simulink model "BESS_F_V_Controle"  (R2017b)
settings: Solver=ode45  StartTime=0.0  StopTime=10  RelTol=1e-3  EnableMultiTasking=on
values from neighbouring files (symbols this model uses):
  beta = beta (k)    [Parameter_2M_DFIG_BESS.m]
  Cbus = 80e-3    (= 0.08)    [Parameter_2M_DFIG_BESS.m]
  Cbus_bess = 15e-3    (= 0.015)    [Parameter_2M_DFIG_BESS.m]
  Cfilter = 80e-3    (= 0.08)    [Parameter_2M_DFIG_BESS.m]
  cp_opt_abs = abs(max(Cp))    [Parameter_2M_DFIG_BESS.m]
  D = 0.1    [Parameter_2M_DFIG_BESS.m]
  f = 60    [Parameter_2M_DFIG_BESS.m]
  Fs = 1.8    [Parameter_2M_DFIG_BESS.m]
  fsw = 4e3    (= 4000)    [Parameter_2M_DFIG_BESS.m]
  J = 90    [Parameter_2M_DFIG_BESS.m]
  ki_id = (wni^2)*Lr*sigma    (= 491.599501999)    [Parameter_2M_DFIG_BESS.m]
  ki_idg = (wnig^2)*Lg    (= 68.6450725305)    [Parameter_2M_DFIG_BESS.m]
  ki_iq = ki_id    (= 491.599501999)    [Parameter_2M_DFIG_BESS.m]
  ki_iqg = ki_idg    (= 68.6450725305)    [Parameter_2M_DFIG_BESS.m]
  ki_v = -300000    [Parameter_2M_DFIG_BESS.m]
  kp_id = (2*wni*sigma*Lr)-Rr    (= 0.5771)    [Parameter_2M_DFIG_BESS.m]
  kp_idg = (2*wnig*Lg)-Rg    (= 0.364153420404)    [Parameter_2M_DFIG_BESS.m]
  kp_iq = kp_id    (= 0.5771)    [Parameter_2M_DFIG_BESS.m]
  kp_iqg = kp_idg    (= 0.364153420404)    [Parameter_2M_DFIG_BESS.m]
  kp_v = -1000    [Parameter_2M_DFIG_BESS.m]
  Kpg = 1/(1.5*Vs*sqrt(2/3))    [Parameter_2M_DFIG_BESS.m]
  Kqg = -Kpg    [Parameter_2M_DFIG_BESS.m]
  lambda_opt = abs(lambda(posicion))    [Parameter_2M_DFIG_BESS.m]
  Lfilter = 483e-6    (= 0.000483)    [Parameter_2M_DFIG_BESS.m]
  Lg = 483e-6    (= 0.000483)    [Parameter_2M_DFIG_BESS.m]
  Lm = 2.5e-3    (= 0.0025)    [Parameter_2M_DFIG_BESS.m]
  Lr = Lm + Lsr    (= 0.002587)    [Parameter_2M_DFIG_BESS.m]
  Ls = Lm + Lsi    (= 0.002587)    [Parameter_2M_DFIG_BESS.m]
  Lsi = 87e-6    (= 8.7e-05)    [Parameter_2M_DFIG_BESS.m]
  N = 100    [Parameter_2M_DFIG_BESS.m]
  p = 2    [Parameter_2M_DFIG_BESS.m]
  Ps = 2e6    (= 2000000)    [Parameter_2M_DFIG_BESS.m]
  Radio = 44    [Parameter_2M_DFIG_BESS.m]
  Rfilter = 20e-3    (= 0.02)    [Parameter_2M_DFIG_BESS.m]
  Rg = 20e-6    (= 2e-05)    [Parameter_2M_DFIG_BESS.m]
  ro = 1.225    [Parameter_2M_DFIG_BESS.m]
  Rr = 2.9e-3    (= 0.0029)    [Parameter_2M_DFIG_BESS.m]
  Rs = 2.6e-3    (= 0.0026)    [Parameter_2M_DFIG_BESS.m]
  sigma = 1- Lm^2/(Ls*Lr)    (= 0.0661284179513)    [Parameter_2M_DFIG_BESS.m]
  Ts = 1/fsw/f    (= 4.16666666667e-06)    [Parameter_2M_DFIG_BESS.m]
  Vbus_ref = 1200    [Parameter_2M_DFIG_BESS.m]
  Vs = 690    [Parameter_2M_DFIG_BESS.m]
undefined symbols (not defined in the file or in its folder): D1, D11, Delta, DiscIntNeverNeededParam, Ion, Lithium, sigbuilder_block
libraries: powerlib x72, powerlib_meascontrol x37, electricdrivelib x1, simulink x1, sps_avr x1
(part 2 of 3)

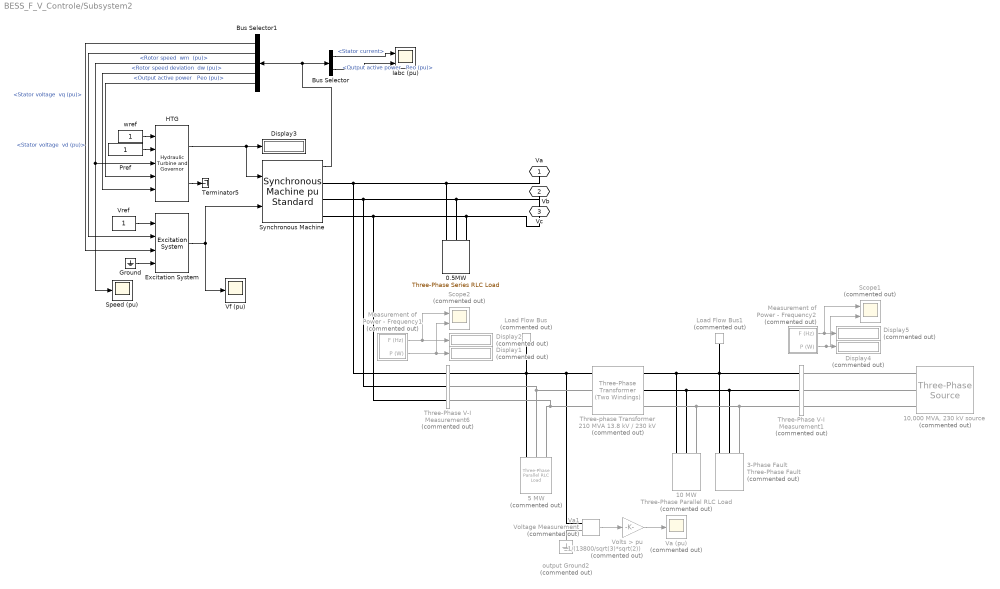
== system BESS_F_V_Controle/Subsystem2 ==
  " Iabc (pu)" : Scope  NumInputPorts=2
  " Speed (pu)" : Scope
  0.5MW : powerlib/Elements/Three-Phase Series RLC Load  LConnTagsString=A|B|C  Configuration=Y (grounded)  NominalVoltage=13800  Vabc=[1e3 1e3 1e3]  Vabcp=[1e3 1e3 1e3]  NominalFrequency=f  UnbalancedPower=off  ActivePower=0.5e6  InductivePower=0  CapacitivePower=0  Pabc=[10e3 9e3 11e3]  QLabc=[100 90 110]  QCabc=[100 90 110]  Pabcp=[10e3 9e3 11e3]  QLabcp=[100 90 110]  QCabcp=[100 90 110]  Measurements=None  LoadType=constant Z
  10 MW : powerlib/Elements/Three-Phase Parallel RLC Load  Commented=on  LConnTagsString=A|B|C  Configuration=Y (grounded)  NominalVoltage=230e3  Vabc=[1e3 1e3 1e3]  Vabcp=[1e3 1e3 1e3]  NominalFrequency=f  UnbalancedPower=off  ActivePower=10000000  InductivePower=0  CapacitivePower=0  Pabc=[10e3 9e3 11e3]  QLabc=[100 90 110]  QCabc=[100 90 110]  Pabcp=[10e3 9e3 11e3]  QLabcp=[100 90 110]  QCabcp=[100 90 110]  Measurements=None  LoadType=constant Z
  "10,000 MVA, 230 kV source" : powerlib/Electrical Sources/Three-Phase Source  Commented=on  InternalConnection=Yg  VoltagePhases=off  Voltage=(230000)*1.00006  PhaseAngle=-0.77547  Voltage_phases=[25e3 25e3 25e3]/sqrt(3)  PhaseAngles_phases=[0 -120 +120]  Frequency=60  NonIdealSource=on  SpecifyImpedance=on  Resistance=0.529  Inductance=0.0140  ShortCircuitLevel=10000e6  BaseVoltage=230e3  XRratio=10  BusType=swing  Pref=0  Qref=0  Prefabc=[10e3, 10e3, 10e3]  Qrefabc=[0, 0, 0]  Qmin=-Inf  Qmax=Inf
  3-Phase Fault : powerlib/Elements/Three-Phase Fault  Commented=on  InitialStates=0  FaultA=on  FaultB=on  FaultC=on  GroundFault=on  SwitchTimes=[ 0.1 0.2]  External=off  SwitchStatus=NaN  FaultResistance=1e-3  GroundResistance=1e-3  SnubberResistance=inf  SnubberCapacitance=inf  Measurements=None
  5 MW : powerlib/Elements/Three-Phase Parallel RLC Load  Commented=on  LConnTagsString=A|B|C  Configuration=Y (grounded)  NominalVoltage=13.8e3  Vabc=[1e3 1e3 1e3]  Vabcp=[1e3 1e3 1e3]  NominalFrequency=60  UnbalancedPower=off  ActivePower=5000000  InductivePower=0  CapacitivePower=0  Pabc=[10e3 9e3 11e3]  QLabc=[100 90 110]  QCabc=[100 90 110]  Pabcp=[10e3 9e3 11e3]  QLabcp=[100 90 110]  QCabcp=[100 90 110]  Measurements=None  LoadType=constant Z
  Bus Selector : BusSelector  OutputSignals="Stator current,Output active power   Peo (pu)"
  Bus Selector1 : BusSelector  OutputSignals="dq0 components.Stator voltage  vq (pu),dq0 components.Stator voltage  vd (pu),Mechanical.Rotor speed  wm  (pu),Mechanical.Rotor speed deviation  dw (pu),Output active power   Peo (pu)"
  Display{1..2,4..5} (4 alike) : Display  Commented=on
  Display3 : Display
  Excitation System : sps_avr/Excitation System  tr=20e-3  reg=[ 300, 0.001 ]  exc=[ 1, 0 ]  tgr=[ 0, 0 ]  damp=[ 0.001, 0.1 ]  sat=[ 0, 0 ]  lim=[ -11.5, 11.5, 0 ]  v0=[1,1.29071]
      settings: SourceProductName=Simscape Power Systems  SourceProductBaseCode=PS
  Ground : Ground
  HTG : powerlib/Machines/Hydraulic Turbine and Governor  sm="[ 10/3  0.07 ]"  gate="[  0.01  0.97518  -0.1  0.1 ]"  reg="[  0.05  1.163  0.105  0  0.01  ]"  hyd="[  0  2.67  ]"  dref=0  po=1
      settings: SourceProductName=Simscape Power Systems  SourceProductBaseCode=PS
  Load Flow Bus : powerlib/Measurements/Load Flow Bus  Commented=on  LConnTagsString=a  Phases=single  Connectors=on one side  ID=B1  Vbase=13.8e3  Vref=1  Vangle=0  VLF=1  VLFb=1  VLFc=1  angleLF=-23.67  angleLFb=0  angleLFc=0
      settings: AttributesFormatString=%<ID>\n%<Vbase>V\n%<VLF>pu\n%<angleLF>deg.  SourceProductName=Simscape Power Systems
  Load Flow Bus1 : powerlib/Measurements/Load Flow Bus  Commented=on  LConnTagsString=a  Phases=single  Connectors=on one side  ID=B2  Vbase=230e3  Vref=1  Vangle=0  VLF=1  VLFb=1  VLFc=1  angleLF=0  angleLFb=0  angleLFc=0
      settings: AttributesFormatString=%<ID>\n%<Vbase>V\n%<VLF>pu\n%<angleLF>deg.  SourceProductName=Simscape Power Systems
  Measurement of Power - Frequency1 : Subsystem  Commented=on
  Measurement of Power - Frequency2 : Subsystem  Commented=on
  Pref : Constant
  Scope1 : Scope  Commented=on  NumInputPorts=2
  Scope2 : Scope  Commented=on  NumInputPorts=2
  "Synchronous Machine " : powerlib/Machines/Synchronous Machine pu Standard  PresetModel=No  MechanicalLoad=Mechanical power Pm  ShowDetailedParameters=on  RotorType=Salient-pole  Units=per unit standard parameters  MeasurementBus=off  NominalParameters="[ 7.5e6  13800   f ]"  Reactances1=[ 31 32 33 34 35 36 37 ]  Reactances2=[ 1.305, 0.296, 0.252, 0.474, 0.243, 0.18 ]  dAxisTimeConstants=Short-circuit  qAxisTimeConstants=Open-circuit  TimeConstants1=[]  TimeConstants2=[]  TimeConstants3=[]  TimeConstants4=[]  TimeConstants5=[ 1.01, 0.053, 0.1 ]  TimeConstants6=[]  TimeConstants7=[]  TimeConstants8=[]  StatorResistance=2.8544e-3  Mechanical=[ 3.2 0 2]  PolePairs=2  InitialConditions=[0 -94.2826 0.750185 0.750185 0.750185 -24.943 -144.943 95.057 1.29071]  SetSaturation=off  Saturation=[0.6404,0.7127,0.8441,0.9214,0.9956,1.082,1.19,1.316,1.457;0.7,0.7698,0.8872,0.9466,0.9969,1.046,1.1,1.151,1.201]  LoadFlowParameters=[1 150000000 0 0]  TsPowergui=0  TsBlock=-1  IterativeModel=Trapezoidal non iterative  IterativeDiscreteModel=Trapezoidal non iterative  BusType=PV  Pref=150000000  Qref=0  Qmin=-Inf  Qmax=Inf  PLF=0  QLF=0
      settings: AttributesFormatString=\n\n  SourceProductName=Simscape Power Systems
  Terminator5 : Terminator
  Three-Phase V-I Measurement1 : powerlib/Measurements/Three-Phase V-I Measurement  Commented=on  VoltageMeasurement=phase-to-ground  SetLabelV=on  LabelV=V_ac_syn_low2  Vpu=off  VpuLL=off  CurrentMeasurement=yes  SetLabelI=on  LabelI=I_ac_syn_low2  Ipu=off  Pbase=100e6  Vbase=500e3  OutputType=Complex  PhasorSimulation=off  PSBequivalent=0
  Three-Phase V-I Measurement6 : powerlib/Measurements/Three-Phase V-I Measurement  Commented=on  VoltageMeasurement=phase-to-ground  SetLabelV=on  LabelV=V_ac_syn_low1  Vpu=off  VpuLL=off  CurrentMeasurement=yes  SetLabelI=on  LabelI=I_ac_syn_low1  Ipu=off  Pbase=100e6  Vbase=500e3  OutputType=Complex  PhasorSimulation=off  PSBequivalent=0
  Three-phase Transformer 210 MVA 13.8 kV / 230 kV : powerlib/Elements/Three-Phase Transformer (Two Windings)  Commented=on  Winding1Connection=Delta (D1)  Winding2Connection=Yg  CoreType=Three single-phase transformers  SetSaturation=off  Hysteresis=off  DataFile='hysteresis'  SetInitialFlux=off  Measurements=None  UNITS=pu  NominalPower=[ 210e6 60 ]  Winding1="[ 13.8e3 0.0027  0.08]"  Winding2=[ 230e3 0.0027 0.08]  Rm=500  Lm=500  L0=0.5  Saturation="[ 0,0  ;  0.005,1.2  ;  1.0,1.4 ]"  InitialFluxes=[ 0.8 , -0.8 , 0.7 ]  MoreParameters=off  BreakLoop=off  DataType=off  TransfoNumber=0
  Va (pu) : Scope  Commented=on
  Va1 : powerlib/Measurements/Voltage Measurement  Tag=PoWeRsYsTeMmEaSuReMeNt  Commented=on  PhasorSimulation=off  OutputType=Magnitude  PSBequivalent=0
  Vf (pu) : Scope
  Volts > pu : Gain  Commented=on  Gain=1/(13800/sqrt(3)*sqrt(2))  SaturateOnIntegerOverflow=on  OutDataTypeStr=Inherit: Same as input  ParamDataTypeStr=Inherit: Same as input
  Vref : Constant
  output Ground2 : powerlib/Elements/Ground  Commented=on  LConnTagsString=a
  wref : Constant
  Va : PMIOPort  Port=1  Side=Left
  Vb : PMIOPort  Port=2  Side=Left
  Vc : PMIOPort  Port=3  Side=Left
  wires:
  Bus Selector1/5 -> HTG/4  "<Output active power   Peo (pu)>"
  HTG/2 -> Terminator5/1
  Bus Selector1/3 -> HTG/3, " Speed (pu)"/1  "<Rotor speed  wm  (pu)>"
  Bus Selector/1 -> " Iabc (pu)"/1  "<Stator current>"
  Bus Selector1/2 -> Excitation System/2  "<Stator voltage  vd (pu)>"
  Ground/1 -> Excitation System/4
  Bus Selector1/1 -> Excitation System/3  "<Stator voltage  vq (pu)>"
  Va1/1 -> Volts > pu/1
  Excitation System/1 -> Vf (pu)/1, "Synchronous Machine "/2
  Bus Selector1/4 -> HTG/5  "<Rotor speed deviation  dw (pu)>"
  Volts > pu/1 -> Va (pu)/1
  Pref/1 -> HTG/2
  wref/1 -> HTG/1
  Vref/1 -> Excitation System/1
  "Synchronous Machine "/1 -> Bus Selector/1, Bus Selector1/1
  Measurement of Power - Frequency1/1(F (Hz)) -> Scope2/1, Display2/1
  Measurement of Power - Frequency1/2(P (W)) -> Scope2/2, Display1/1
  Bus Selector/2 -> " Iabc (pu)"/2  "<Output active power   Peo (pu)>"
  HTG/1 -> "Synchronous Machine "/1, Display3/1
  Measurement of Power - Frequency2/1(F (Hz)) -> Scope1/1, Display5/1
  Measurement of Power - Frequency2/2(P (W)) -> Scope1/2, Display4/1
  connections:
  Va1/LConn1 -- Three-Phase V-I Measurement6/RConn1 -- 5 MW/LConn1 -- Load Flow Bus/LConn1 -- Three-phase Transformer 210 MVA 13.8 kV / 230 kV/LConn1
  5 MW/LConn3 -- Three-Phase V-I Measurement6/RConn3 -- Three-phase Transformer 210 MVA 13.8 kV / 230 kV/LConn3
  10 MW/LConn2 -- Three-phase Transformer 210 MVA 13.8 kV / 230 kV/RConn2 -- Three-Phase V-I Measurement1/LConn2 -- 3-Phase Fault/LConn2
  Load Flow Bus1/LConn1 -- Three-phase Transformer 210 MVA 13.8 kV / 230 kV/RConn1 -- 10 MW/LConn1 -- Three-Phase V-I Measurement1/LConn1 -- 3-Phase Fault/LConn1
  3-Phase Fault/LConn3 -- Three-Phase V-I Measurement1/LConn3 -- Three-phase Transformer 210 MVA 13.8 kV / 230 kV/RConn3 -- 10 MW/LConn3
  5 MW/LConn2 -- Three-Phase V-I Measurement6/RConn2 -- Three-phase Transformer 210 MVA 13.8 kV / 230 kV/LConn2
  output Ground2/LConn1 -- Va1/LConn2
  0.5MW/LConn1 -- Three-Phase V-I Measurement6/LConn1 -- "Synchronous Machine "/RConn1 -- Va/RConn1
  Vb/RConn1 -- "Synchronous Machine "/RConn2 -- Three-Phase V-I Measurement6/LConn2 -- 0.5MW/LConn2
  0.5MW/LConn3 -- "Synchronous Machine "/RConn3 -- Three-Phase V-I Measurement6/LConn3 -- Vc/RConn1
  Three-Phase V-I Measurement1/RConn1 -- "10,000 MVA, 230 kV source"/RConn1
  Three-Phase V-I Measurement1/RConn2 -- "10,000 MVA, 230 kV source"/RConn2
  Three-Phase V-I Measurement1/RConn3 -- "10,000 MVA, 230 kV source"/RConn3

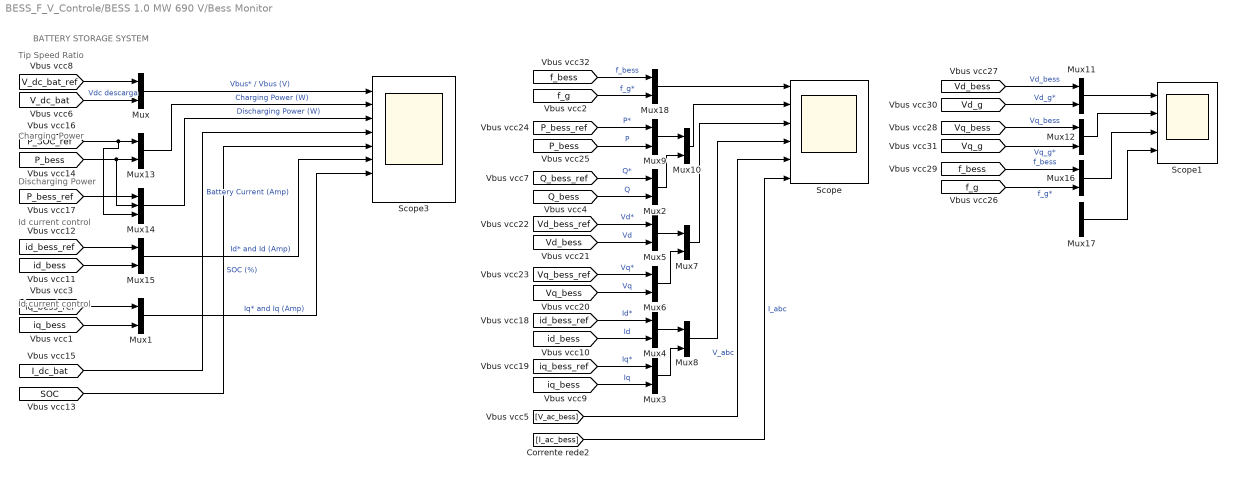
== system BESS_F_V_Controle/BESS 1.0 MW 690 V/Bess Monitor ==
  note: BATTERY STORAGE SYSTEM
  note: Tip Speed Ratio
  note: Charging Power
  note: Discharging Power
  note: Id current control
  note: Id current control
  Mux{,1..13,15..18} (18 alike) : Mux  Inputs=2
  Mux14 : Mux  Inputs=3
  Scope : Scope  NumInputPorts=6
  Scope1 : Scope  NumInputPorts=4
  Scope3 : Scope  NumInputPorts=8
  wires:
  [P_bess_ref] -> Mux14/1
  Mux13/1 -> Scope3/2  "Charging Power (W)"
  [P_SOC_ref] -> Mux14/3, Mux13/1
  [P_bess] -> Mux14/2, Mux13/2
  [id_bess_ref] -> Mux15/1
  [V_dc_bat_ref] -> Mux/1
  Mux/1 -> Scope3/1  "Vbus* / Vbus (V)"
  [id_bess] -> Mux15/2
  Mux14/1 -> Scope3/3  "Discharging Power (W)"
  [SOC] -> Scope3/5  "SOC (%)"
  [I_dc_bat] -> Scope3/4  "Battery Current (Amp)"
  Mux15/1 -> Scope3/6  "Id* and Id (Amp)"
  [V_dc_bat] -> Mux/2  "Vdc descarga"
  [iq_bess] -> Mux1/2
  [iq_bess_ref] -> Mux1/1
  Mux1/1 -> Scope3/7  "Iq* and Iq (Amp)"
  [Q_bess_ref] -> Mux2/1  "Q*"
  [Q_bess] -> Mux2/2  "Q"
  [iq_bess_ref] -> Mux3/1  "Iq*"
  [id_bess] -> Mux4/2  "Id"
  [iq_bess] -> Mux3/2  "Iq"
  [id_bess_ref] -> Mux4/1  "Id*"
  [Vq_bess_ref] -> Mux6/1  "Vq*"
  [Vq_bess] -> Mux6/2  "Vq"
  Mux4/1 -> Mux8/1
  Mux6/1 -> Mux7/2
  Mux5/1 -> Mux7/1
  Mux7/1 -> Scope/3
  Mux3/1 -> Mux8/2
  Mux8/1 -> Scope/4
  [V_ac_bess] -> Scope/5  "V_abc"
  [I_ac_bess] -> Scope/6  "I_abc"
  [P_bess_ref] -> Mux9/1  "P*"
  [P_bess] -> Mux9/2  "P"
  Mux9/1 -> Mux10/1
  Mux2/1 -> Mux10/2
  Mux10/1 -> Scope/2
  [Vd_bess] -> Mux5/2  "Vd"
  [Vd_bess_ref] -> Mux5/1  "Vd*"
  [Vq_g] -> Mux12/2  "Vq_g*"
  [Vq_bess] -> Mux12/1  "Vq_bess"
  [Vd_bess] -> Mux11/1  "Vd_bess"
  Mux17/1 -> Scope1/4
  [Vd_g] -> Mux11/2  "Vd_g*"
  Mux11/1 -> Scope1/1
  Mux16/1 -> Scope1/3
  [f_bess] -> Mux16/1  "f_bess"
  [f_g] -> Mux16/2  "f_g*"
  Mux12/1 -> Scope1/2
  [f_bess] -> Mux18/1  "f_bess"
  [f_g] -> Mux18/2  "f_g*"
  Mux18/1 -> Scope/1

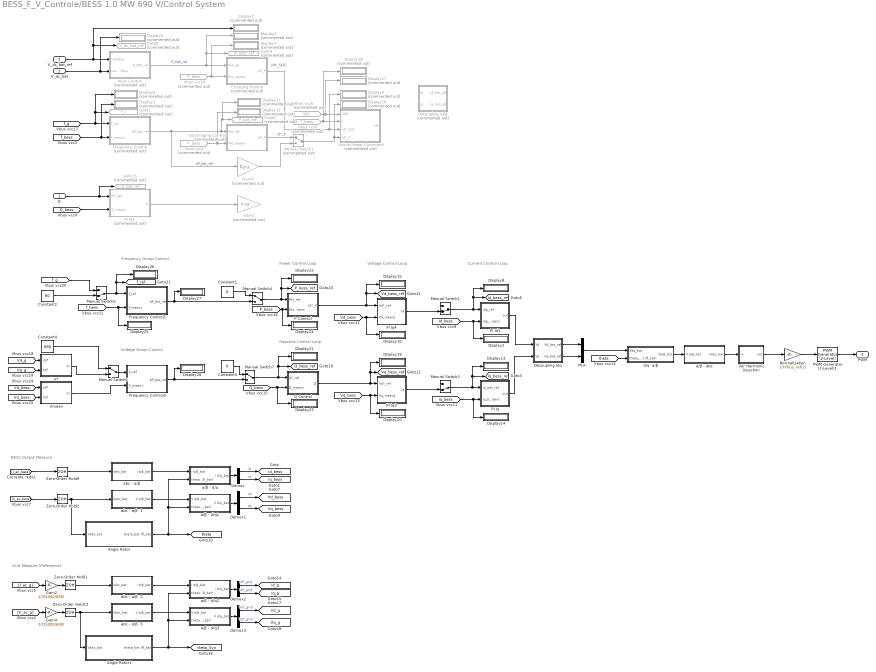
== system BESS_F_V_Controle/BESS 1.0 MW 690 V/Control System ==
  note: BESS Output Measure
  note: Id*_SOC
  note: Grid Measure (Reference)
  note: Current Control Loop
  note: Voltage Control Loop
  note: Power Control Loop
  note: Frequency Droop Control
  note: Voltage Droop Control
  note: Reactive Control Loop
  Q : Inport
  V_dc_bat : Inport  Port=2
  V_dc_bat_ref : Inport  Port=3
  " Angle Rotor" : Subsystem
  " Angle Rotor1" : Subsystem
  3er Harmonic Inyection : Subsystem
  Active Power Command : Subsystem  Commented=on
  Charging Control : Subsystem  Commented=on
  Constant1 : Constant  Value=0
  Constant2 : Constant  Value=60
  Constant3 : Constant  Value=0
  Constant4 : Constant  Value=690
  Decoupling Idq : Subsystem
  Decoupling Vdq : Subsystem  Commented=on
  Demux{,1..3} (4 alike) : Demux  Outputs=2
  Dischraging Control : Subsystem  Commented=on
  Display{1,3..7,9..12,17..18} (12 alike) : Display  Commented=on
  Display{2,8,13..16,19..28} (16 alike) : Display
  Frequency Control : Subsystem  Commented=on
  Frequency Control1 : Subsystem
  Frequency Control2 : Subsystem
  Gain1 : Gain  Commented=on  Gain=Kqg
  Gain2 : Gain  Gain=1/(25000/690)
  Gain3 : Gain  Commented=on  Gain=Kpg
  Gain4 : Gain  Gain=1/(25000/690)
  Goto13 : Goto  Commented=on  GotoTag=Q_bat_ref  TagVisibility=global
  Goto2 : Goto  Commented=on  GotoTag=f_r  TagVisibility=global
  Goto4 : Goto  Commented=on  GotoTag=P_SOC_ref  TagVisibility=global
  Goto6 : Goto  Commented=on  GotoTag=P_bat_ref  TagVisibility=global
  Goto8 : Goto  Commented=on  GotoTag=V_dc_bat_ref  TagVisibility=global
  Manual Switch1 : ManualSwitch  Commented=on
  Manual Switch2 : ManualSwitch  CurrentSetting=0
  Manual Switch3 : ManualSwitch  CurrentSetting=0
  Manual Switch4 : ManualSwitch
  Manual Switch5 : ManualSwitch  CurrentSetting=0
  Manual Switch6 : ManualSwitch
  Manual Switch7 : ManualSwitch
  Mux : Mux  Inputs=2
  Normalization : Gain  Gain=1/(Vbus_ref/2)
  P Control : Subsystem
  PI Id1 : Subsystem
  PI Iq : Subsystem
  PI Iq1 : Subsystem  Commented=on
  PI Iq3 : Subsystem
  PI Iq4 : Subsystem
  PWM Generator (2-Level)1 : powerlib_meascontrol/Pulse & Signal Generators/PWM Generator (2-Level)  ModulatorType=Three-phase bridge (6 pulses)  ModulatorMode=Unsynchronized  Fc=fsw  Pc=0  nF=27  MinMax="[ -1  1 ]"  SamplingTechnique=Natural  ModulatingSignals=off  m=0.8  Freq=60  Phase=0  Ts=0  ShowCarrierOutport=off
      settings: SourceProductName=Simscape Power Systems
  Q Control : Subsystem
  V* : Subsystem
  Vbus Control : Subsystem  Commented=on
  Vbus vcc1 : From  Commented=on  GotoTag=P_bess  TagVisibility=global
  Vbus vcc10 : From  Commented=on  GotoTag=P_bess  TagVisibility=global
  Vbus vcc6 : From  Commented=on  GotoTag=f_bess  TagVisibility=global
  Vbus vcc8 : From  Commented=on  GotoTag=SOC  TagVisibility=global
  Vmean : Subsystem
  Zero-Order Hold{1..2,9,13} (4 alike) : ZeroOrderHold  SampleTime=1/fsw
  "abc - α/β  " : Subsystem
  abc - α/β  1 : Subsystem
  abc - α/β  2 : Subsystem
  abc - α/β  3 : Subsystem
  "d/q  α/β " : Subsystem
  α/β - abc : Subsystem
  α/β - d/q : Subsystem
  α/β - d/q1 : Subsystem
  α/β - d/q2 : Subsystem
  α/β - d/q3 : Subsystem
  PWM : Outport
  tag scope: P_bess_ref=global, Q_bess_ref=global, Vd_bess=global, Vd_bess_ref=global, Vd_g=global, Vq_bess=global, Vq_bess_ref=global, Vq_g=global, f_ref=global, id_bess=global, id_bess_ref=global, id_g=global, iq_bess=global, iq_bess_ref=global, iq_g=global, theta=global, theta_Syn=global
  wires:
  PWM Generator (2-Level)1/1 -> PWM/1
  α/β - d/q/1(i d/q_bat) -> Demux/1
  Zero-Order Hold2/1 -> " Angle Rotor"/1(Vabc_bat), abc - α/β  1/1(Vabc_bat)
  α/β - abc/1(Vabc_bat) -> 3er Harmonic Inyection/1(in)
  Zero-Order Hold9/1 -> "abc - α/β  "/1(iabc_bat)
  "d/q  α/β "/1("Vα/β_bat ") -> α/β - abc/1(V α/β_bat)
  "abc - α/β  "/1(i α/β_bat) -> α/β - d/q/1(i α/β_bat)
  3er Harmonic Inyection/1(out) -> Normalization/1
  PI Id1/1(out) -> Decoupling Idq/1(Vd)
  PI Iq/1("out ") -> Decoupling Idq/2(Vq)
  Normalization/1 -> PWM Generator (2-Level)1/1
  V_dc_bat/1 -> Display6/1, Vbus Control/2("means Vbus ")
  [f_g] -> Frequency Control/1(f_ref), Goto2/1, Display5/1
  Vbus vcc1/1 -> Display12/1, Dischraging Control/2("Pot_means ")
  [f_bess] -> Display1/1, Frequency Control/2(f_means)
  Vbus vcc6/1 -> Active Power Command/2(f), Display18/1
  Vbus vcc8/1 -> Active Power Command/1(SOC), Display17/1
  V_dc_bat_ref/1 -> Goto8/1, Display7/1, Vbus Control/1("ref Vbus ")
  Charging Control/1(Id*_P) -> Display9/1, Active Power Command/3(Id*_SOC)
  Vbus Control/1(P_SOC_ref) -> Goto4/1, Display4/1, Charging Control/1("Pot_ref ")  "P_SOC_ref"
  Vbus vcc10/1 -> Charging Control/2("Pot_means "), Display3/1
  [Q_bess] -> PI Iq1/2(Q_means)
  Demux1/1 -> [Vd_bess]  "Vd"
  abc - α/β  1/1(V α/β_bat) -> α/β - d/q1/1(V α/β_bat)
  α/β - d/q1/1(V d/q_bat) -> Demux1/1
  Demux1/2 -> [Vq_bess]  "Vq"
  Q/1 -> Goto13/1, PI Iq1/1(Q*_ref)
  Mux/1 -> "d/q  α/β "/1(Vdq_bat)
  PI Iq1/1("Q ") -> Gain1/1
  Decoupling Idq/1(" Vd_bat_ref") -> Mux/1
  Decoupling Idq/2(" Vq_bat_ref") -> Mux/2
  " Angle Rotor"/1(theta_bat (θ_bat)) -> α/β - d/q1/2(theta_bat (θ_bat)), α/β - d/q/2(theta_bat (θ_bat)), [theta]
  Demux/1 -> [id_bess]  "id"
  Demux/2 -> [iq_bess]  "iq"
  [theta] -> "d/q  α/β "/2(theta_bat (θ_bat))
  [id_bess] -> PI Id1/2(idg_means), Display2/1
  [iq_bess] -> Display14/1, PI Iq/2(iq_bat_means)
  P Control/1(Id*_P) -> Display15/1, [Vd_bess_ref], PI Iq4/1(Vd*_ref)
  [Vd_bess] -> Display16/1, PI Iq4/2(Vd_means)
  [Vq_bess] -> Display20/1, PI Iq3/2(Vq_means)
  Q Control/1("Q ") -> Display19/1, [Vq_bess_ref], PI Iq3/1(Vq*_ref)
  Frequency Control/1("ΔP_bat_ref ") -> Dischraging Control/1("Pot_ref "), Display11/1, Goto6/1, Gain3/1  "ΔP_bat_ref"
  Dischraging Control/1(Id*_P) -> Manual Switch1/1  "Id*_P"
  Gain3/1 -> Manual Switch1/2
  Manual Switch1/1 -> Active Power Command/4(Id*_P), Display10/1
  Demux3/2 -> [Vq_g]  "Vq*_grid"
  Demux3/1 -> [Vd_g]  "Vd*_grid"
  abc - α/β  3/1(V α/β_bat) -> α/β - d/q3/1(V α/β_bat)
  abc - α/β  2/1(i α/β_bat) -> α/β - d/q2/1(i α/β_bat)
  " Angle Rotor1"/1(theta_bat (θ_bat)) -> α/β - d/q3/2(theta_bat (θ_bat)), α/β - d/q2/2(theta_bat (θ_bat)), [theta_Syn]
  Demux2/1 -> [id_g]  "id*_grid"
  Demux2/2 -> [iq_g]  "iq*_grid"
  α/β - d/q2/1(i d/q_bat) -> Demux2/1
  α/β - d/q3/1(V d/q_bat) -> Demux3/1
  [I_ac_g] -> Gain2/1
  Gain2/1 -> Zero-Order Hold1/1
  [V_ac_g] -> Gain4/1
  Gain4/1 -> Zero-Order Hold13/1
  Zero-Order Hold1/1 -> abc - α/β  2/1(iabc_bat)
  Zero-Order Hold13/1 -> " Angle Rotor1"/1(Vabc_bat), abc - α/β  3/1(Vabc_bat)
  [I_ac_bess] -> Zero-Order Hold9/1
  [V_ac_bess] -> Zero-Order Hold2/1
  [P_bess] -> Display24/1, P Control/2("Pot_means ")
  Manual Switch2/1 -> Display8/1, [id_bess_ref], PI Id1/1(idg_ref)
  Manual Switch3/1 -> Display13/1, [iq_bess_ref], PI Iq/1(iq_bat_ref)
  PI Iq4/1("Id ") -> Manual Switch2/2
  PI Iq3/1("Iq ") -> Manual Switch3/2
  [f_bess] -> Display25/1, Frequency Control1/2(f_means)
  Manual Switch4/1 -> [P_bess_ref], Display22/1, P Control/1("Pot_ref ")
  Frequency Control1/1("ΔP_bat_ref ") -> Manual Switch4/2, Display27/1
  Constant1/1 -> Manual Switch4/1
  Manual Switch5/1 -> Display26/1, [f_ref], Frequency Control1/1(f_ref)
  [f_g] -> Manual Switch5/1
  Constant2/1 -> Manual Switch5/2
  [Vq_g] -> V*/2(Vq*)
  [Vd_g] -> V*/1(Vd*)
  [Vd_bess] -> Vmean/1(Vd*)
  [Vq_bess] -> Vmean/2(Vq*)
  Frequency Control2/1("ΔP_bat_ref ") -> Manual Switch7/2, Display28/1
  Manual Switch6/1 -> Frequency Control2/1(V_ref)
  Constant4/1 -> Manual Switch6/1
  [Q_bess] -> Display23/1, Q Control/2(Q_means)
  Manual Switch7/1 -> [Q_bess_ref], Display21/1, Q Control/1(Q*_ref)
  Constant3/1 -> Manual Switch7/1
  V*/1("V* ") -> Manual Switch6/2
  Vmean/1("V* ") -> Frequency Control2/2(V_means)

== system BESS_F_V_Controle/BESS 1.0 MW 690 V/Measurement of Power - Frequency ==
  PLL (3ph)1 : powerlib_meascontrol/PLL/PLL (3ph)  Fmin=45  Par_Init=[0, f]  ParK=[180, 3200, 1]  TcD=1e-4  MaxRateChangeFreq=12  FilterCutOffFreq=25  Ts=0  AGC=on
  "Power (3ph, Instantaneous)1" : powerlib_meascontrol/Measurements/Power (3ph, Instantaneous)
      settings: SourceProductName=Simscape Power Systems
  F (Hz) : Outport
  P (W) : Outport  Port=2
  Q (VAR) : Outport  Port=3
  Angle (0) : Outport  Port=4
  tag scope: P_bess=global, Q_bess=global, f_bess=global, wt_mean=global
  wires:
  [V_ac_bess] -> "Power (3ph, Instantaneous)1"/1, PLL (3ph)1/1
  "Power (3ph, Instantaneous)1"/1 -> P (W)/1, [P_bess]  "Pot"
  PLL (3ph)1/1 -> F (Hz)/1, [f_bess]
  [I_ac_bess] -> "Power (3ph, Instantaneous)1"/2
  "Power (3ph, Instantaneous)1"/2 -> Q (VAR)/1, [Q_bess]
  PLL (3ph)1/2 -> Angle (0)/1, [wt_mean]

== system BESS_F_V_Controle/BESS 1.0 MW 690 V/Measurement of Power - Frequency1 ==
  PLL (3ph)1 : powerlib_meascontrol/PLL/PLL (3ph)  Fmin=45  Par_Init=[0, f]  ParK=[180, 3200, 1]  TcD=1e-4  MaxRateChangeFreq=12  FilterCutOffFreq=25  Ts=0  AGC=on
  "Power (3ph, Instantaneous)1" : powerlib_meascontrol/Measurements/Power (3ph, Instantaneous)
      settings: SourceProductName=Simscape Power Systems
  P (W) : Outport
  f (Hz) : Outport  Port=2
  tag scope: f_g=global
  wires:
  [V_ac_g] -> PLL (3ph)1/1, "Power (3ph, Instantaneous)1"/1
  "Power (3ph, Instantaneous)1"/1 -> P (W)/1  "Pot"
  [I_ac_g] -> "Power (3ph, Instantaneous)1"/2
  PLL (3ph)1/1 -> [f_g], f (Hz)/1

== system BESS_F_V_Controle/BESS 1.0 MW 690 V/Measurement of Power - Frequency2 ==
  "Power (3ph, Instantaneous)1" : powerlib_meascontrol/Measurements/Power (3ph, Instantaneous)
      settings: SourceProductName=Simscape Power Systems
  P (W) : Outport
  wires:
  [I_ac_line_1] -> "Power (3ph, Instantaneous)1"/2
  "Power (3ph, Instantaneous)1"/1 -> P (W)/1  "Pot"
  [V_ac_line_1] -> "Power (3ph, Instantaneous)1"/1

== system BESS_F_V_Controle/BESS 1.0 MW 690 V/Measurement of Power - Frequency3 ==
  "Power (3ph, Instantaneous)1" : powerlib_meascontrol/Measurements/Power (3ph, Instantaneous)
      settings: SourceProductName=Simscape Power Systems
  P (W) : Outport
  wires:
  [V_ac_line_2_1] -> "Power (3ph, Instantaneous)1"/1
  "Power (3ph, Instantaneous)1"/1 -> P (W)/1  "Pot"
  [I_ac_line_2_1] -> "Power (3ph, Instantaneous)1"/2

== system BESS_F_V_Controle/BESS 1.0 MW 690 V/Subsystem1 ==
  In1 : Inport
  Bus Selector : BusSelector  OutputSignals=SOC (%),Current (A),Voltage (V)
  tag scope: I_dc_bat=global, SOC=global, V_dc_bat=global
  wires:
  Bus Selector/3 -> [V_dc_bat]  "<Voltage (V)>"
  Bus Selector/1 -> [SOC]  "<SOC (%)>"
  In1/1 -> Bus Selector/1
  Bus Selector/2 -> [I_dc_bat]  "<Current (A)>"

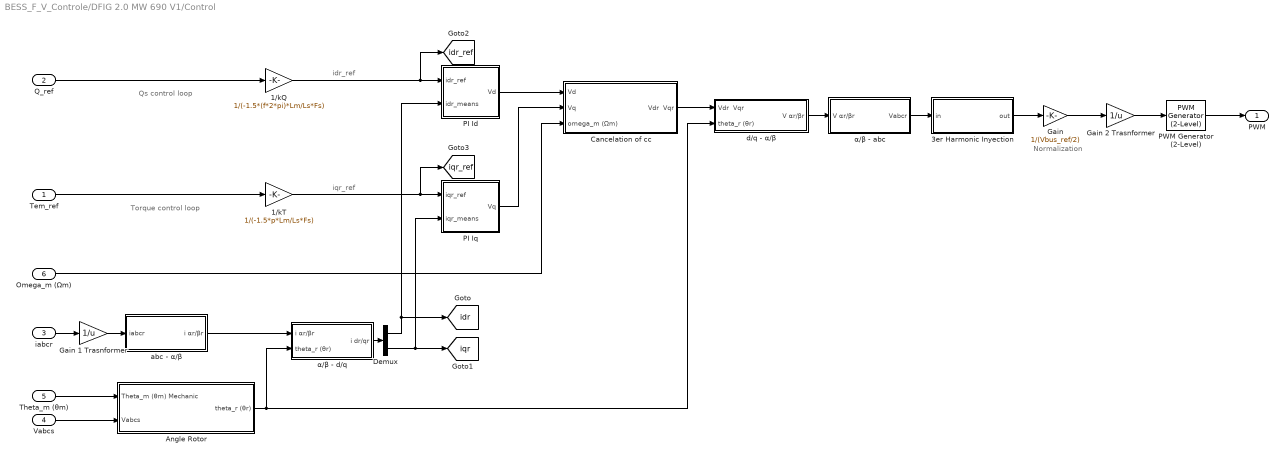
== system BESS_F_V_Controle/DFIG 2.0 MW 690 V1/Control ==
  note: Normalization
  note: Torque control loop
  note: iqr_ref
  note: idr_ref
  note: Qs control loop
  Tem_ref : Inport
  Q_ref : Inport  Port=2
  iabcr : Inport  Port=3
  Vabcs : Inport  Port=4
  Theta_m (θm) : Inport  Port=5
  "Omega_m (Ωm) " : Inport  Port=6
  " Angle Rotor" : Subsystem
  1/kQ : Gain  Gain=1/(-1.5*(f*2*pi)*Lm/Ls*Fs)
  1/kT : Gain  Gain=1/(-1.5*p*Lm/Ls*Fs)
  3er Harmonic Inyection : Subsystem
  Cancelation of cc : Subsystem
  Demux : Demux  Outputs=2
  Gain : Gain  Gain=1/(Vbus_ref/2)
  Gain 1 Trasnformer : Gain  Gain=1/u
  Gain 2 Trasnformer : Gain  Gain=1/u
  PI Id : Subsystem
  PI Iq : Subsystem
  PWM Generator (2-Level) : powerlib_meascontrol/Pulse & Signal Generators/PWM Generator (2-Level)  ModulatorType=Three-phase bridge (6 pulses)  ModulatorMode=Unsynchronized  Fc=fsw  Pc=0  nF=27  MinMax="[ -1  1 ]"  SamplingTechnique=Natural  ModulatingSignals=off  m=0.8  Freq=60  Phase=0  Ts=0  ShowCarrierOutport=off
      settings: SourceProductName=Simscape Power Systems
  "abc - α/β " : Subsystem
  d/q - α/β : Subsystem
  α/β - abc : Subsystem
  α/β - d/q : Subsystem
  PWM : Outport
  tag scope: idr=global, idr_ref=global, iqr=global, iqr_ref=global
  wires:
  α/β - abc/1(Vabcr) -> 3er Harmonic Inyection/1(in)
  d/q - α/β/1(V αr/βr) -> α/β - abc/1(V αr/βr)
  iabcr/1 -> Gain 1 Trasnformer/1
  "abc - α/β "/1(i αr/βr) -> α/β - d/q/1(i αr/βr)
  3er Harmonic Inyection/1(out) -> Gain/1
  Theta_m (θm)/1 -> " Angle Rotor"/1(Theta_m (θm) Mechanic)
  Vabcs/1 -> " Angle Rotor"/2(Vabcs)
  " Angle Rotor"/1(theta_r (θr)) -> d/q - α/β/2(theta_r (θr)), α/β - d/q/2(theta_r (θr))
  PI Id/1(Vd) -> Cancelation of cc/1(Vd)
  PI Iq/1(Vq) -> Cancelation of cc/2(Vq)
  α/β - d/q/1(i dr/qr) -> Demux/1
  Demux/2 -> PI Iq/2(iqr_means), [iqr]
  Demux/1 -> PI Id/2(idr_means), [idr]
  1/kT/1 -> [iqr_ref], PI Iq/1(iqr_ref)
  Q_ref/1 -> 1/kQ/1
  Cancelation of cc/1(Vdr  Vqr) -> d/q - α/β/1(Vdr  Vqr)
  Gain/1 -> Gain 2 Trasnformer/1
  Gain 1 Trasnformer/1 -> "abc - α/β "/1(iabcr)
  Gain 2 Trasnformer/1 -> PWM Generator (2-Level)/1
  PWM Generator (2-Level)/1 -> PWM/1
  Tem_ref/1 -> 1/kT/1
  "Omega_m (Ωm) "/1 -> Cancelation of cc/3(omega_m (Ωm))
  1/kQ/1 -> [idr_ref], PI Id/1(idr_ref)

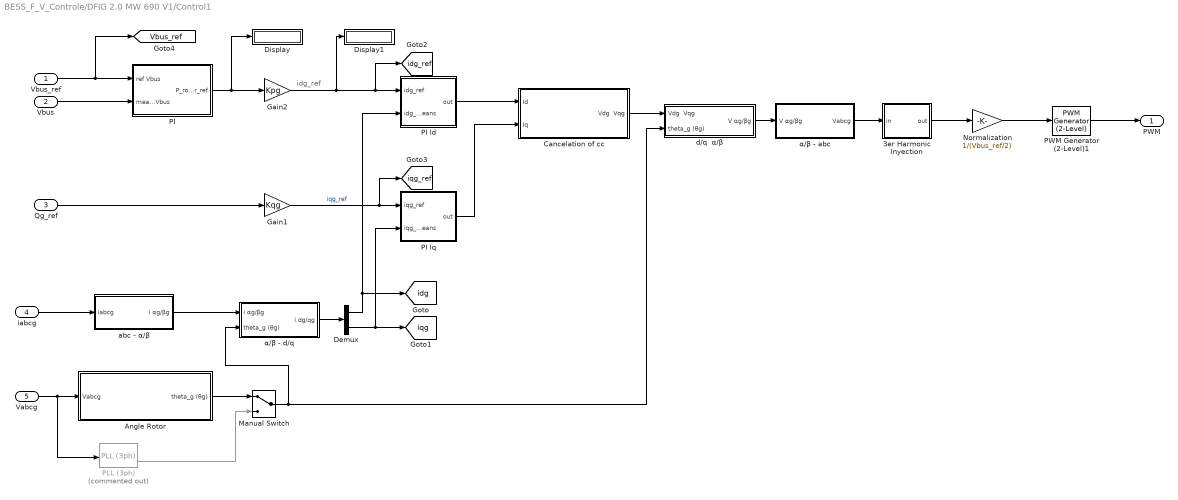
== system BESS_F_V_Controle/DFIG 2.0 MW 690 V1/Control1 ==
  note: idg_ref
  Vbus_ref : Inport
  Vbus : Inport  Port=2
  Qg_ref : Inport  Port=3
  iabcg : Inport  Port=4
  "Vabcg " : Inport  Port=5
  " Angle Rotor" : Subsystem
  3er Harmonic Inyection : Subsystem
  Cancelation of cc : Subsystem
  Demux : Demux  Outputs=2
  Display : Display
  Display1 : Display
  Gain1 : Gain  Gain=Kqg
  Gain2 : Gain  Gain=Kpg
  Manual Switch : ManualSwitch
  Normalization : Gain  Gain=1/(Vbus_ref/2)
  PI : Subsystem
  PI Id : Subsystem
  PI Iq : Subsystem
  PLL (3ph) : powerlib_meascontrol/PLL/PLL (3ph)  Commented=on  Fmin=45  Par_Init=[0, 60]  ParK=[180, 3200, 1]  TcD=1e-4  MaxRateChangeFreq=12  FilterCutOffFreq=25  Ts=0  AGC=on
      link override Model/abc to dq0: Alignment=Aligned with phase A axis
  PWM Generator (2-Level)1 : powerlib_meascontrol/Pulse & Signal Generators/PWM Generator (2-Level)  ModulatorType=Three-phase bridge (6 pulses)  ModulatorMode=Unsynchronized  Fc=fsw  Pc=0  nF=27  MinMax="[ -1  1 ]"  SamplingTechnique=Natural  ModulatingSignals=off  m=0.8  Freq=60  Phase=0  Ts=0  ShowCarrierOutport=off
      settings: SourceProductName=Simscape Power Systems
  "abc - α/β  " : Subsystem
  "d/q  α/β " : Subsystem
  α/β - abc : Subsystem
  α/β - d/q : Subsystem
  PWM : Outport
  tag scope: Vbus_ref=global, idg=global, idg_ref=global, iqg=global, iqg_ref=global
  wires:
  Normalization/1 -> PWM Generator (2-Level)1/1
  Cancelation of cc/1(Vdg  Vqg) -> "d/q  α/β "/1(Vdg  Vqg)
  Gain1/1 -> PI Iq/1(iqg_ref), [iqg_ref]  "iqg_ref"
  Demux/1 -> PI Id/2(idg_means), [idg]
  Demux/2 -> PI Iq/2(iqg_means), [iqg]
  PI Iq/1(out) -> Cancelation of cc/2(Iq)
  PI Id/1(out) -> Cancelation of cc/1(Id)
  3er Harmonic Inyection/1(out) -> Normalization/1
  "abc - α/β  "/1(i αg/βg) -> α/β - d/q/1(i αg/βg)
  "d/q  α/β "/1(V αg/βg) -> α/β - abc/1(V αg/βg)
  iabcg/1 -> "abc - α/β  "/1(iabcg)
  Vbus_ref/1 -> [Vbus_ref], PI/1("ref Vbus ")
  Gain2/1 -> Display1/1, [idg_ref], PI Id/1(idg_ref)
  Vbus/1 -> PI/2("means Vbus ")
  Qg_ref/1 -> Gain1/1
  α/β - abc/1(Vabcg) -> 3er Harmonic Inyection/1(in)
  "Vabcg "/1 -> " Angle Rotor"/1("Vabcg "), PLL (3ph)/1
  PI/1(P_rotor_ref) -> Display/1, Gain2/1
  " Angle Rotor"/1(theta_g (θg)) -> Manual Switch/1
  Manual Switch/1 -> "d/q  α/β "/2(theta_g (θg)), α/β - d/q/2(theta_g (θg))
  α/β - d/q/1(i dg/qg) -> Demux/1
  PLL (3ph)/2 -> Manual Switch/2
  PWM Generator (2-Level)1/1 -> PWM/1

== system BESS_F_V_Controle/DFIG 2.0 MW 690 V1/MPPT ==
  note: Zone 2: MPPT with Vw 5 - 11
  Omega_m : Inport
  Display1 : Display
  Display2 : Display
  Gearbox Ratio Generator Torque (-)1 : Gain  Gain=-1/N
  Gearbox Ratio1 : Gain  Gain=1/N
  Kopt : Gain  Gain=0.5*ro*pi*(Radio)^5/(lambda_opt)^3*cp_opt_abs
  Product2 : Product  Inputs=**  SaturateOnIntegerOverflow=on  InputSameDT=on  OutDataTypeStr=Inherit: Same as first input
  omega^2 : Fcn  Expr=(u[1])^2
  Tem_ref : Outport
  "Pot_ref " : Outport  Port=2
  wires:
  Gearbox Ratio1/1 -> Product2/2, omega^2/1
  omega^2/1 -> Kopt/1
  Kopt/1 -> Product2/1, Gearbox Ratio Generator Torque (-)1/1
  Product2/1 -> "Pot_ref "/1, Display1/1  "Pt"
  Gearbox Ratio Generator Torque (-)1/1 -> Display2/1, Tem_ref/1
  Omega_m/1 -> Gearbox Ratio1/1

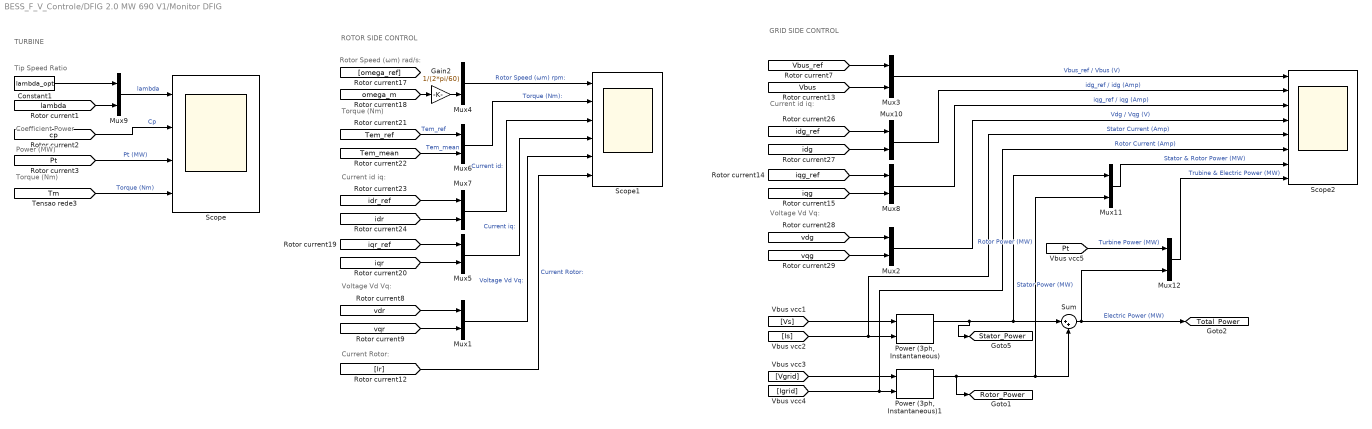
== system BESS_F_V_Controle/DFIG 2.0 MW 690 V1/Monitor DFIG ==
  note: ROTOR SIDE CONTROL
  note: Torque (Nm)
  note: Current id iq:
  note: Rotor Speed (ωm) rad/s:
  note: Voltage Vd Vq:
  note: TURBINE
  note: Torque (Nm)
  note: Power (MW)
  note: Coefficient Power
  note: Tip Speed Ratio
  note: GRID SIDE CONTROL
  note: Current id iq:
  note: Voltage Vd Vq:
  note: Current Rotor:
  Constant1 : Constant  Value=lambda_opt
  Gain2 : Gain  Gain=1/(2*pi/60)
  Mux{1..12} (12 alike) : Mux  Inputs=2
  "Power (3ph, Instantaneous)" : powerlib_meascontrol/Measurements/Power (3ph, Instantaneous)
      settings: SourceProductName=Simscape Power Systems
  "Power (3ph, Instantaneous)1" : powerlib_meascontrol/Measurements/Power (3ph, Instantaneous)
      settings: SourceProductName=Simscape Power Systems
  Scope : Scope  NumInputPorts=4
  Scope1 : Scope  NumInputPorts=6
  Scope2 : Scope  NumInputPorts=8
  Sum : Sum  Inputs=|++
  tag scope: Rotor_Power=global, Stator_Power=global, Total_Power=global
  wires:
  [iqr_ref] -> Mux5/1
  [iqr] -> Mux5/2
  [idr] -> Mux7/2
  [idr_ref] -> Mux7/1
  [vdr] -> Mux1/1
  [vqr] -> Mux1/2
  [vqg] -> Mux2/2
  [vdg] -> Mux2/1
  [idg_ref] -> Mux10/1
  [idg] -> Mux10/2
  [iqg] -> Mux8/2
  [iqg_ref] -> Mux8/1
  [Tem_ref] -> Mux6/1  "Tem_ref"
  [Vbus] -> Mux3/2
  [Vbus_ref] -> Mux3/1
  [cp] -> Scope/2  "Cp"
  [Pt] -> Scope/3  "Pt (MW)"
  [Tm] -> Scope/4  "Torque (Nm)"
  Mux4/1 -> Scope1/1  "Rotor Speed (ωm) rpm:"
  Mux6/1 -> Scope1/2  "Torque (Nm):"
  Mux7/1 -> Scope1/3  "Current id:"
  Mux5/1 -> Scope1/4  "Current iq:"
  Mux1/1 -> Scope1/5  "Voltage Vd Vq:"
  [Ir] -> Scope1/6  "Current Rotor:"
  [omega_m] -> Gain2/1
  Gain2/1 -> Mux4/2
  Mux3/1 -> Scope2/1  "Vbus_ref / Vbus (V)"
  Mux10/1 -> Scope2/2  "idg_ref / idg (Amp)"
  Mux8/1 -> Scope2/3  "iqg_ref / iqg (Amp)"
  Mux2/1 -> Scope2/4  "Vdg / Vqg (V)"
  [lambda] -> Mux9/2
  Constant1/1 -> Mux9/1
  Mux9/1 -> Scope/1  "lambda"
  [Tem_mean] -> Mux6/2  "Tem_mean"
  [Vs] -> "Power (3ph, Instantaneous)"/1
  [Vgrid] -> "Power (3ph, Instantaneous)1"/1
  [Igrid] -> "Power (3ph, Instantaneous)1"/2, Scope2/6  "Rotor Current (Amp)"
  [Is] -> "Power (3ph, Instantaneous)"/2, Scope2/5  "Stator Current (Amp)"
  "Power (3ph, Instantaneous)"/1 -> [Stator_Power], Mux11/1, Sum/1  "Stator Power (MW)"
  "Power (3ph, Instantaneous)1"/1 -> [Rotor_Power], Sum/2, Mux11/2  "Rotor Power (MW)"
  Sum/1 -> [Total_Power], Mux12/2  "Electric Power (MW)"
  Mux11/1 -> Scope2/7  "Stator & Rotor Power (MW)"
  [Pt] -> Mux12/1  "Turbine Power (MW)"
  Mux12/1 -> Scope2/8  "Trubine & Electric Power (MW)"

== system BESS_F_V_Controle/DFIG 2.0 MW 690 V1/Signal Builder ==
  Demux : Demux  Tag=STV Demux  Outputs=1
  FromWs : FromWorkspace  Tag=STV FromWs  VariableName=tuvar  SampleTime=0
      SigBuilderData=|
      | common.afterFinalStr = 'Extrapolate'
      | common.sampleTime = 0
      | dataSet.timeRange = [0 20]
      | dataSet.name = 'Group 1'
      | sbobj.Groups.Name = 'Group 1'
      | sbobj.Groups.Signals.Name = 'Signal 1'
      | sbobj.Groups.Signals.XData = [0 1.5 4.8 5 5.2 5.44 5.7 6.08 6.5 6.84 7.18 7.62 8 8.42 8.98 9.48 10 10.4 10.88 11.36 11.8 12.32 12.88 13.38 14.1 14.74 15.28 15.86 16.32 16.86 17.5 18.1 18.62 19.32 20]
      | sbobj.Groups.Signals.YData = [0 11.5 11.5471428571 11.4 10.8 10.752 10.7 10.81875 11.05 11.4 11.5 11.6 11.65 11.65 11.5 11.3 11.35 11.35 11.45 11.35 11.15 11.35 11.5 11.4859550562 11.55 11.5228813559 11.5 11.4754237288 11.4559322034 11.4330508475 11.4059322034 11.3805084746 11.3584745763 11.3288135593 11.3]
      | sbobj.Groups.TimeRange = [0 20]
  Signal 1 : Outport  Tag=STV Outport
  wires:
  Demux/1 -> Signal 1/1
  FromWs/1 -> Demux/1

== system BESS_F_V_Controle/DFIG 2.0 MW 690 V1/Subsystem ==
  In1 : Inport
  Bus Selector : BusSelector  OutputSignals=Mechanical.Rotor angle thetam (rad),Mechanical.Rotor speed (wm),Mechanical.Electromagnetic torque Te (N*m)
  tag scope: Tem_mean=global, omega_m=global, tita_m=global
  wires:
  Bus Selector/2 -> [omega_m]  "<Rotor speed (wm)>"
  In1/1 -> Bus Selector/1
  Bus Selector/1 -> [tita_m]  "<Rotor angle thetam (rad)>"
  Bus Selector/3 -> [Tem_mean]  "<Electromagnetic torque Te (N*m)>"

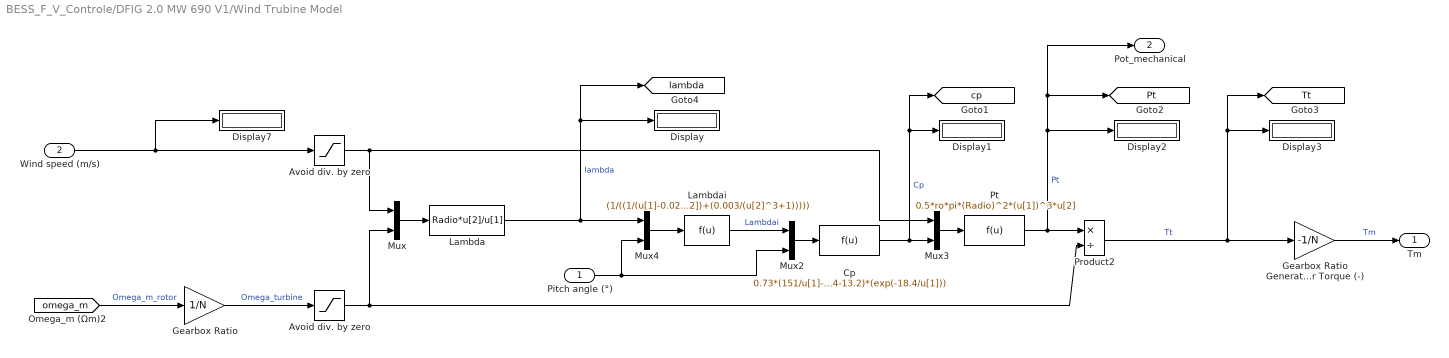
== system BESS_F_V_Controle/DFIG 2.0 MW 690 V1/Wind Trubine Model ==
  Pitch angle (°) : Inport
  Wind speed (m/s) : Inport  Port=2
  Avoid div. by zero : Saturate  UpperLimit=inf  LowerLimit=eps
  "Avoid div. by zero " : Saturate  UpperLimit=inf  LowerLimit=eps
  Cp : Fcn  Expr=0.73*(151/u[1]-0.58*u[2]-0.002*u[2]^2.14-13.2)*(exp(-18.4/u[1]))
  Display{,1..3,7} (5 alike) : Display
  Gearbox Ratio : Gain  Gain=1/N
  Gearbox Ratio Generator Torque (-) : Gain  Gain=-1/N
  Lambda : Fcn  Expr=Radio*u[2]/u[1]
  Lambdai : Fcn  Expr=(1/((1/(u[1]-0.02*u[2])+(0.003/(u[2]^3+1)))))
  Mux{,2..4} (4 alike) : Mux  Inputs=2
  Product2 : Product  Inputs=*/  SaturateOnIntegerOverflow=on  InputSameDT=on  OutDataTypeStr=Inherit: Same as first input
  Pt : Fcn  Expr=0.5*ro*pi*(Radio)^2*(u[1])^3*u[2]
  Tm : Outport
  Pot_mechanical : Outport  Port=2
  tag scope: Pt=global, Tt=global, cp=global, lambda=global
  wires:
  "Avoid div. by zero "/1 -> Product2/2, Mux/2
  Avoid div. by zero/1 -> Mux/1, Mux3/1
  [omega_m] -> Gearbox Ratio/1  "Omega_m_rotor"
  Mux3/1 -> Pt/1
  Cp/1 -> Display1/1, [cp], Mux3/2  "Cp"
  Mux/1 -> Lambda/1
  Mux2/1 -> Cp/1
  Product2/1 -> Display3/1, [Tt], Gearbox Ratio Generator Torque (-)/1  "Tt"
  Pt/1 -> Display2/1, Pot_mechanical/1, [Pt], Product2/1  "Pt"
  Gearbox Ratio/1 -> "Avoid div. by zero "/1  "Omega_turbine"
  Wind speed (m/s)/1 -> Display7/1, Avoid div. by zero/1
  Lambdai/1 -> Mux2/1  "Lambdai"
  Mux4/1 -> Lambdai/1
  Gearbox Ratio Generator Torque (-)/1 -> Tm/1  "Tm"
  Pitch angle (°)/1 -> Mux2/2, Mux4/2
  Lambda/1 -> Display/1, [lambda], Mux4/1  "lambda"

== system BESS_F_V_Controle/Subsystem2/Measurement of Power - Frequency1 ==
  PLL (3ph)1 : powerlib_meascontrol/PLL/PLL (3ph)  Fmin=45  Par_Init=[0, f]  ParK=[180, 3200, 1]  TcD=1e-4  MaxRateChangeFreq=12  FilterCutOffFreq=25  Ts=0  AGC=on
  "Power (3ph, Instantaneous)1" : powerlib_meascontrol/Measurements/Power (3ph, Instantaneous)
      settings: SourceProductName=Simscape Power Systems
  F (Hz) : Outport
  P (W) : Outport  Port=2
  wires:
  [I_ac_syn_low1] -> "Power (3ph, Instantaneous)1"/2
  PLL (3ph)1/1 -> F (Hz)/1
  "Power (3ph, Instantaneous)1"/1 -> P (W)/1  "Pot"
  [V_ac_syn_low1] -> PLL (3ph)1/1, "Power (3ph, Instantaneous)1"/1

== system BESS_F_V_Controle/Subsystem2/Measurement of Power - Frequency2 ==
  PLL (3ph)1 : powerlib_meascontrol/PLL/PLL (3ph)  Fmin=45  Par_Init=[0, f]  ParK=[180, 3200, 1]  TcD=1e-4  MaxRateChangeFreq=12  FilterCutOffFreq=25  Ts=0  AGC=on
  "Power (3ph, Instantaneous)1" : powerlib_meascontrol/Measurements/Power (3ph, Instantaneous)
      settings: SourceProductName=Simscape Power Systems
  F (Hz) : Outport
  P (W) : Outport  Port=2
  wires:
  [I_ac_syn_low2] -> "Power (3ph, Instantaneous)1"/2
  PLL (3ph)1/1 -> F (Hz)/1
  "Power (3ph, Instantaneous)1"/1 -> P (W)/1  "Pot"
  [V_ac_syn_low2] -> PLL (3ph)1/1, "Power (3ph, Instantaneous)1"/1

== system BESS_F_V_Controle/BESS 1.0 MW 690 V/Control System/ Angle Rotor ==
  note: V α/β_bat
  Vabc_bat : Inport
  " abc - αβ " : Subsystem
  Demux : Demux  Outputs=2
  Manual Switch : ManualSwitch
  PLL (3ph) : powerlib_meascontrol/PLL/PLL (3ph)  Commented=on  Fmin=45  Par_Init=[0, 60]  ParK=[180, 3200, 1]  TcD=1e-4  MaxRateChangeFreq=12  FilterCutOffFreq=25  Ts=0  AGC=on
      link override Model/abc to dq0: Alignment=Aligned with phase A axis
  θv=tan^(-1) (Vβ/Vα) : Trigonometry  Operator=atan2
  theta_bat (θ_bat) : Outport
  wires:
  Demux/2 -> θv=tan^(-1) (Vβ/Vα)/1
  Demux/1 -> θv=tan^(-1) (Vβ/Vα)/2
  " abc - αβ "/1("V α/β_bat ") -> Demux/1
  Vabc_bat/1 -> PLL (3ph)/1, " abc - αβ "/1(Vabc_bat)
  PLL (3ph)/2 -> Manual Switch/2
  θv=tan^(-1) (Vβ/Vα)/1 -> Manual Switch/1
  Manual Switch/1 -> theta_bat (θ_bat)/1

== system BESS_F_V_Controle/BESS 1.0 MW 690 V/Control System/ Angle Rotor1 ==
  note: V α/β_bat
  Vabc_bat : Inport
  " abc - αβ " : Subsystem
  Demux : Demux  Outputs=2
  Manual Switch : ManualSwitch
  PLL (3ph) : powerlib_meascontrol/PLL/PLL (3ph)  Commented=on  Fmin=45  Par_Init=[0, 60]  ParK=[180, 3200, 1]  TcD=1e-4  MaxRateChangeFreq=12  FilterCutOffFreq=25  Ts=0  AGC=on
      link override Model/abc to dq0: Alignment=Aligned with phase A axis
  θv=tan^(-1) (Vβ/Vα) : Trigonometry  Operator=atan2
  theta_bat (θ_bat) : Outport
  wires:
  Demux/2 -> θv=tan^(-1) (Vβ/Vα)/1
  Demux/1 -> θv=tan^(-1) (Vβ/Vα)/2
  " abc - αβ "/1("V α/β_bat ") -> Demux/1
  Vabc_bat/1 -> PLL (3ph)/1, " abc - αβ "/1(Vabc_bat)
  PLL (3ph)/2 -> Manual Switch/2
  θv=tan^(-1) (Vβ/Vα)/1 -> Manual Switch/1
  Manual Switch/1 -> theta_bat (θ_bat)/1

== system BESS_F_V_Controle/BESS 1.0 MW 690 V/Control System/3er Harmonic Inyection ==
  in : Inport
  Gain : Gain  Gain=-0.5
  MinMax : MinMax
  MinMax1 : MinMax  Function=max
  Scope : Scope
  Sum : Sum  Inputs=|++
  Sum1 : Sum  Inputs=|++
  out : Outport
  wires:
  in/1 -> Sum1/1, MinMax1/1, MinMax/1
  MinMax/1 -> Sum/1
  MinMax1/1 -> Sum/2
  Sum1/1 -> out/1
  Sum/1 -> Gain/1
  Gain/1 -> Scope/1, Sum1/2

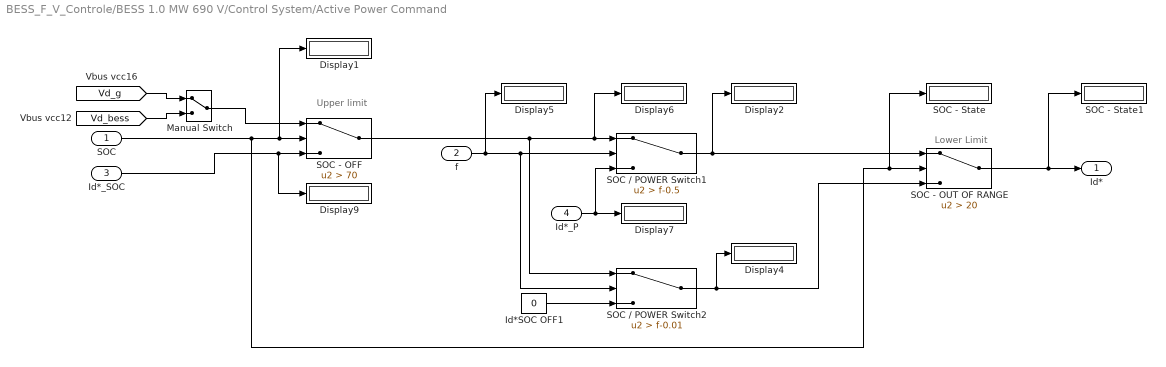
== system BESS_F_V_Controle/BESS 1.0 MW 690 V/Control System/Active Power Command ==
  note: Lower Limit
  note: Upper limit
  SOC : Inport
  f : Inport  Port=2
  Id*_SOC : Inport  Port=3
  Id*_P : Inport  Port=4
  Display{1..2,4..7,9} (7 alike) : Display
  Id*SOC OFF1 : Constant  Value=0
  Manual Switch : ManualSwitch
  SOC - OFF : Switch  Criteria=u2 > Threshold  Threshold=70
  SOC - OUT OF RANGE : Switch  Criteria=u2 > Threshold  Threshold=20
  SOC - State : Display
  SOC - State1 : Display
  SOC / POWER Switch1 : Switch  Criteria=u2 > Threshold  Threshold=f-0.5
  SOC / POWER Switch2 : Switch  Criteria=u2 > Threshold  Threshold=f-0.01
  Id* : Outport
  wires:
  SOC / POWER Switch1/1 -> SOC - OUT OF RANGE/1, Display2/1
  f/1 -> Display5/1, SOC / POWER Switch2/2, SOC / POWER Switch1/2
  Id*_P/1 -> SOC / POWER Switch1/3, Display7/1
  SOC - OFF/1 -> SOC / POWER Switch2/1, SOC / POWER Switch1/1, Display6/1
  Id*_SOC/1 -> Display9/1, SOC - OFF/3
  SOC / POWER Switch2/1 -> Display4/1, SOC - OUT OF RANGE/3
  SOC - OUT OF RANGE/1 -> SOC - State1/1, Id*/1
  Id*SOC OFF1/1 -> SOC / POWER Switch2/3
  SOC/1 -> SOC - State/1, SOC - OUT OF RANGE/2, Display1/1, SOC - OFF/2
  Manual Switch/1 -> SOC - OFF/1
  [Vd_bess] -> Manual Switch/2
  [Vd_g] -> Manual Switch/1

== system BESS_F_V_Controle/BESS 1.0 MW 690 V/Control System/Charging Control ==
  "Pot_ref " : Inport
  "Pot_means " : Inport  Port=2
  Discrete-Time Integrator1 : DiscreteIntegrator  gainval=1  SampleTime=1/fsw  LimitOutput=on  UpperSaturationLimit=1200  LowerSaturationLimit=-1200  ICPrevOutput=DiscIntNeverNeededParam  ICPrevScaledInput=DiscIntNeverNeededParam
  Display6 : Display
  Error : Display
  Gain1 : Gain  Gain=Kpg
  Gain2 : Gain  Gain=Kpg
  Gain3 : Gain  Gain=0.03
  Mean : Display
  Mux : Mux  Inputs=3
  Ref : Display
  Sat : Display
  Sat1 : Display
  Saturation : Saturate  UpperLimit=1200  LowerLimit=-1200
  Scope : Scope
  Sum2 : Sum  Inputs=|+-
  Sum3 : Sum  Inputs=|++
  Id*_P : Outport
  wires:
  Sum2/1 -> Error/1, Mux/3, Gain2/1, Gain3/1
  Gain1/1 -> Display6/1
  Gain2/1 -> Sum3/1
  Sum3/1 -> Saturation/1
  Gain3/1 -> Discrete-Time Integrator1/1
  Discrete-Time Integrator1/1 -> Sat1/1, Sum3/2
  Mux/1 -> Scope/1
  "Pot_ref "/1 -> Mux/1, Ref/1, Gain1/1, Sum2/1
  "Pot_means "/1 -> Mux/2, Mean/1, Sum2/2
  Saturation/1 -> Sat/1, Id*_P/1

== system BESS_F_V_Controle/BESS 1.0 MW 690 V/Control System/Decoupling Idq ==
  Vd : Inport
  Vq : Inport  Port=2
  Fcn : Fcn  Expr=u[1]-u[4]*Lfilter*(2*pi*f)
  Fcn1 : Fcn  Expr=u[2]+u[3]*Lfilter*(2*pi*f)
  Mux1 : Mux
  Sum : Sum  Inputs=|++
  Sum1 : Sum  Inputs=|++
  " Vd_bat_ref" : Outport
  " Vq_bat_ref" : Outport  Port=2
  tag scope: Vd=global, Vq=global
  wires:
  Vd/1 -> Mux1/1
  Vq/1 -> Mux1/2
  Mux1/1 -> Fcn1/1, Fcn/1
  [id_bess] -> Mux1/3
  [iq_bess] -> Mux1/4
  Sum1/1 -> [Vq], " Vq_bat_ref"/1
  Fcn1/1 -> Sum1/1  "Vq*"
  Fcn/1 -> Sum/1  "Vd*"
  Sum/1 -> [Vd], " Vd_bat_ref"/1
  [Vd_bess] -> Sum/2
  [Vq_bess] -> Sum1/2

== system BESS_F_V_Controle/BESS 1.0 MW 690 V/Control System/Decoupling Vdq ==
  Id : Inport
  Iq : Inport  Port=2
  Fcn : Fcn  Expr=u[1]-u[4]*Cfilter*(2*pi*f)
  Fcn1 : Fcn  Expr=u[2]+u[3]*Cfilter*(2*pi*f)
  Mux1 : Mux
  Sum : Sum  Inputs=|++
  Sum1 : Sum  Inputs=|++
  " Id_bat_ref" : Outport
  " Iq_bat_ref" : Outport  Port=2
  tag scope: Id=global, Iq=global
  wires:
  Id/1 -> Mux1/1
  Iq/1 -> Mux1/2
  Mux1/1 -> Fcn1/1, Fcn/1
  [Vd_bess] -> Mux1/3
  [Vq_bess] -> Mux1/4
  Fcn/1 -> Sum/1  "Id*"
  Sum/1 -> [Id], " Id_bat_ref"/1
  Fcn1/1 -> Sum1/1  "Iq*"
  Sum1/1 -> [Iq], " Iq_bat_ref"/1
  [iq_bess] -> Sum1/2
  [id_bess] -> Sum/2

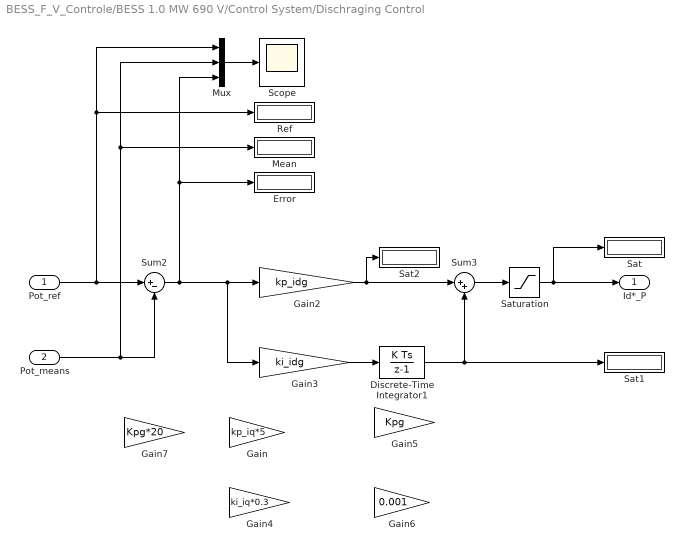
== system BESS_F_V_Controle/BESS 1.0 MW 690 V/Control System/Dischraging Control ==
  "Pot_ref " : Inport
  "Pot_means " : Inport  Port=2
  Discrete-Time Integrator1 : DiscreteIntegrator  gainval=1  SampleTime=1/fsw  LimitOutput=on  UpperSaturationLimit=690  LowerSaturationLimit=-690  ICPrevOutput=DiscIntNeverNeededParam  ICPrevScaledInput=DiscIntNeverNeededParam
  Error : Display
  Gain : Gain  Gain=kp_iq*5
  Gain2 : Gain  Gain=kp_idg
  Gain3 : Gain  Gain=ki_idg
  Gain4 : Gain  Gain=ki_iq*0.3
  Gain5 : Gain  Gain=Kpg
  Gain6 : Gain  Gain=0.001
  Gain7 : Gain  Gain=Kpg*20
  Mean : Display
  Mux : Mux  Inputs=3
  Ref : Display
  Sat : Display
  Sat1 : Display
  Sat2 : Display
  Saturation : Saturate  UpperLimit=1850  LowerLimit=-1850
  Scope : Scope
  Sum2 : Sum  Inputs=|+-
  Sum3 : Sum  Inputs=|++
  Id*_P : Outport
  wires:
  Saturation/1 -> Id*_P/1, Sat/1
  "Pot_means "/1 -> Sum2/2, Mean/1, Mux/2
  "Pot_ref "/1 -> Sum2/1, Ref/1, Mux/1
  Mux/1 -> Scope/1
  Discrete-Time Integrator1/1 -> Sum3/2, Sat1/1
  Gain3/1 -> Discrete-Time Integrator1/1
  Sum3/1 -> Saturation/1
  Gain2/1 -> Sat2/1, Sum3/1
  Sum2/1 -> Gain3/1, Gain2/1, Mux/3, Error/1

== system BESS_F_V_Controle/BESS 1.0 MW 690 V/Control System/Frequency Control ==
  note: Δf = f_ref - f_means
  note: R = (Δf/fo)/(ΔP/Po)*100
  note: ΔP = 1/fo* Δf * 1/R * 100 * Po
  f_ref : Inport
  f_means : Inport  Port=2
  Dead Zone1 : DeadZone  LowerValue=-0.12*1/f  UpperValue=0.02*1/f  SaturateOnIntegerOverflow=on
  Droop : Gain  Gain=1/(3.5)*100
  Error : Display
  Mean : Display
  Mux : Mux  Inputs=3
  Ref : Display
  Saturation : Saturate  UpperLimit=1  LowerLimit=0
  Saturation1 : Saturate  UpperLimit=1000000  LowerLimit=0
  Scope : Scope
  Scope1 : Scope
  Sum : Sum  Inputs=|+-
  "pu_Pot " : Gain  Gain=2.6e6
  pu_f : Gain  Gain=1/f
  pu_f2 : Gain  Gain=1/f
  ΔP_bat_ref : Display
  ΔP_bat_ref1 : Display
  "ΔP_bat_ref " : Outport
  wires:
  Mux/1 -> Scope/1
  f_ref/1 -> pu_f/1
  f_means/1 -> pu_f2/1
  Droop/1 -> Saturation/1
  Sum/1 -> Dead Zone1/1, Mux/3, Error/1
  Saturation/1 -> ΔP_bat_ref1/1, "pu_Pot "/1
  pu_f/1 -> Sum/1, Mux/1, Ref/1
  pu_f2/1 -> Sum/2, Mux/2, Mean/1
  "pu_Pot "/1 -> Saturation1/1
  Saturation1/1 -> Scope1/1, ΔP_bat_ref/1, "ΔP_bat_ref "/1
  Dead Zone1/1 -> Droop/1

== system BESS_F_V_Controle/BESS 1.0 MW 690 V/Control System/Frequency Control1 ==
  note: Δf = f_ref - f_means
  note: R = (Δf/fo)/(ΔP/Po)*100
  note: ΔP = 1/fo* Δf * 1/R * 100 * Po
  f_ref : Inport
  f_means : Inport  Port=2
  Dead Zone1 : DeadZone  LowerValue=-0.12*1/f  UpperValue=0.02*1/f  SaturateOnIntegerOverflow=on
  Droop : Gain  Gain=1/(3.5)*100
  Error : Display
  Mean : Display
  Mux : Mux  Inputs=3
  Ref : Display
  Saturation : Saturate  UpperLimit=1  LowerLimit=0
  Saturation1 : Saturate  UpperLimit=1.5e6  LowerLimit=0
  Scope : Scope
  Scope1 : Scope
  Sum : Sum  Inputs=|+-
  "pu_Pot " : Gain  Gain=1.5e6
  pu_f : Gain  Gain=1/f
  pu_f2 : Gain  Gain=1/f
  ΔP_bat_ref : Display
  ΔP_bat_ref1 : Display
  "ΔP_bat_ref " : Outport
  wires:
  Mux/1 -> Scope/1
  f_ref/1 -> pu_f/1
  f_means/1 -> pu_f2/1
  Droop/1 -> Saturation/1
  Sum/1 -> Dead Zone1/1, Mux/3, Error/1
  Saturation/1 -> ΔP_bat_ref1/1, "pu_Pot "/1
  pu_f/1 -> Sum/1, Mux/1, Ref/1
  pu_f2/1 -> Sum/2, Mux/2, Mean/1
  "pu_Pot "/1 -> Saturation1/1
  Saturation1/1 -> Scope1/1, ΔP_bat_ref/1, "ΔP_bat_ref "/1
  Dead Zone1/1 -> Droop/1

== system BESS_F_V_Controle/BESS 1.0 MW 690 V/Control System/Frequency Control2 ==
  note: ΔV = 1/Qo* ΔV * 1/R * 100 * Qo
  note: R = (Δf/fo)/(ΔP/Po)*100
  note: ΔQ = Q_ref - Q_means
  V_ref : Inport
  V_means : Inport  Port=2
  Dead Zone1 : DeadZone  LowerValue=-0.12*1/f  UpperValue=0.02*1/f  SaturateOnIntegerOverflow=on
  Droop : Gain  Gain=1/(3.5)*100
  Error : Display
  Mean : Display
  Mux : Mux  Inputs=3
  Ref : Display
  Saturation1 : Saturate  UpperLimit=1.5e6  LowerLimit=0
  Scope : Scope
  Scope1 : Scope
  Sum : Sum  Inputs=|+-
  pu_Q1 : Gain  Gain=1/100
  ΔP_bat_ref : Display
  ΔP_bat_ref1 : Display
  "ΔP_bat_ref " : Outport
  wires:
  Dead Zone1/1 -> Droop/1
  Saturation1/1 -> "ΔP_bat_ref "/1, ΔP_bat_ref/1, Scope1/1
  Droop/1 -> Saturation1/1, ΔP_bat_ref1/1
  V_means/1 -> Mean/1, Mux/2, Sum/2
  V_ref/1 -> Ref/1, Mux/1, Sum/1
  Sum/1 -> Error/1, Mux/3, Dead Zone1/1
  Mux/1 -> Scope/1

== system BESS_F_V_Controle/BESS 1.0 MW 690 V/Control System/P Control ==
  "Pot_ref " : Inport
  "Pot_means " : Inport  Port=2
  Discrete-Time Integrator1 : DiscreteIntegrator  gainval=1  SampleTime=1/fsw  LimitOutput=on  UpperSaturationLimit=1.5e6  LowerSaturationLimit=-1.5e6  ICPrevOutput=DiscIntNeverNeededParam  ICPrevScaledInput=DiscIntNeverNeededParam
  Error : Display
  Gain1 : Gain  Gain=kp_idg*0.5
  Gain4 : Gain  Gain=ki_idg
  Gain5 : Gain  Gain=Kpg
  Mean : Display
  Mux : Mux  Inputs=3
  Ref : Display
  Sat : Display
  Sat1 : Display
  Sat2 : Display
  Saturation : Saturate  UpperLimit=1.5e6  LowerLimit=-1.5e6
  Scope : Scope
  Sum2 : Sum  Inputs=|+-
  Sum3 : Sum  Inputs=|++
  Id*_P : Outport
  wires:
  Sum2/1 -> Error/1, Mux/3, Gain4/1, Gain1/1
  Gain1/1 -> Sum3/1, Sat2/1
  Sum3/1 -> Saturation/1
  Gain4/1 -> Discrete-Time Integrator1/1
  Discrete-Time Integrator1/1 -> Sat1/1, Sum3/2
  Mux/1 -> Scope/1
  "Pot_ref "/1 -> Sum2/1, Mux/1, Ref/1
  "Pot_means "/1 -> Mux/2, Mean/1, Sum2/2
  Saturation/1 -> Gain5/1, Sat/1
  Gain5/1 -> Id*_P/1

== system BESS_F_V_Controle/BESS 1.0 MW 690 V/Control System/PI Id1 ==
  idg_ref : Inport
  idg_means : Inport  Port=2
  Discrete-Time Integrator : DiscreteIntegrator  SampleTime=1/fsw  LimitOutput=on  UpperSaturationLimit=Vbus_ref/sqrt(3)*5  LowerSaturationLimit=-Vbus_ref/sqrt(3)*5  ICPrevOutput=DiscIntNeverNeededParam  ICPrevScaledInput=DiscIntNeverNeededParam
  Error : Display
  Gain : Gain  Gain=kp_idg
  Gain1 : Gain  Gain=ki_idg
  Mean : Display
  Mux : Mux  Inputs=3
  Ref : Display
  Sat : Display
  Sat 1 : Display
  Saturation : Saturate  UpperLimit=Vbus_ref/sqrt(3)*6  LowerLimit=-Vbus_ref/sqrt(3)*6
  Scope : Scope
  Sum : Sum  Inputs=|+-
  Sum1 : Sum  Inputs=|++
  out : Outport
  wires:
  Saturation/1 -> Sat/1, out/1
  Sum1/1 -> Saturation/1
  Discrete-Time Integrator/1 -> Sat 1/1, Sum1/2
  Gain1/1 -> Discrete-Time Integrator/1
  Gain/1 -> Sum1/1
  idg_means/1 -> Mean/1, Mux/2, Sum/2
  idg_ref/1 -> Ref/1, Mux/1, Sum/1
  Sum/1 -> Gain/1, Gain1/1, Mux/3, Error/1
  Mux/1 -> Scope/1

== system BESS_F_V_Controle/BESS 1.0 MW 690 V/Control System/PI Iq ==
  iq_bat_ref : Inport
  iq_bat_means : Inport  Port=2
  Discrete-Time Integrator : DiscreteIntegrator  SampleTime=1/fsw  LimitOutput=on  UpperSaturationLimit=Vbus_ref/sqrt(3)  LowerSaturationLimit=-Vbus_ref/sqrt(3)  ICPrevOutput=DiscIntNeverNeededParam  ICPrevScaledInput=DiscIntNeverNeededParam
  Error : Display
  Gain : Gain  Gain=kp_iqg
  Gain1 : Gain  Gain=ki_iqg
  Mean : Display
  Mux : Mux  Inputs=3
  Ref : Display
  Sat : Display
  Sat 1 : Display
  Saturation : Saturate  UpperLimit=Vbus_ref/sqrt(3)  LowerLimit=-Vbus_ref/sqrt(3)
  Scope : Scope
  Sum : Sum  Inputs=|+-
  Sum1 : Sum  Inputs=|++
  "out " : Outport
  wires:
  Mux/1 -> Scope/1
  Sum/1 -> Gain1/1, Gain/1, Error/1, Mux/3
  iq_bat_ref/1 -> Mux/1, Ref/1, Sum/1
  iq_bat_means/1 -> Mux/2, Mean/1, Sum/2
  Saturation/1 -> "out "/1, Sat/1
  Gain/1 -> Sum1/1
  Gain1/1 -> Discrete-Time Integrator/1
  Discrete-Time Integrator/1 -> Sum1/2, Sat 1/1
  Sum1/1 -> Saturation/1
